simulink subsystem "Subsystem"  (R2024b)
settings: Solver=VariableStepAuto  StartTime=0.0  StopTime=10.0  RelTol=1e-3
settings Model: Creator=samueljoseph  LastModifiedBy=samueljoseph

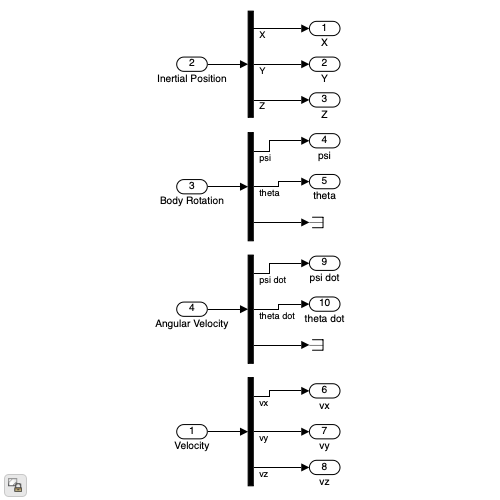
[thumbnail: Simulink's stored preview of the top-level diagram]
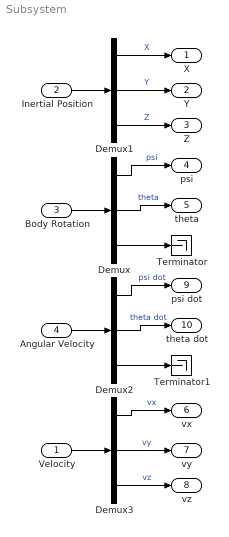
== system Subsystem ==
  Velocity : Inport
  Inertial Position : Inport  Port=2
  Body Rotation : Inport  Port=3
  Angular Velocity : Inport  Port=4
  Demux{,1..3} (4 alike) : Demux  Outputs=3
  Terminator : Terminator
  Terminator1 : Terminator
  X : Outport
  Y : Outport  Port=2
  Z : Outport  Port=3
  psi : Outport  Port=4
  theta : Outport  Port=5
  vx : Outport  Port=6
  vy : Outport  Port=7
  vz : Outport  Port=8
  psi dot : Outport  Port=9
  theta dot : Outport  Port=10
  wires:
  Demux3/3 -> vz/1  "vz"
  Demux3/2 -> vy/1  "vy"
  Demux1/2 -> Y/1  "Y"
  Demux1/1 -> X/1  "X"
  Demux2/3 -> Terminator1/1
  Demux3/1 -> vx/1  "vx"
  Demux2/2 -> theta dot/1  "theta dot"
  Demux1/3 -> Z/1  "Z"
  Demux/2 -> theta/1  "theta"
  Body Rotation/1 -> Demux/1
  Demux/1 -> psi/1  "psi"
  Velocity/1 -> Demux3/1
  Demux2/1 -> psi dot/1  "psi dot"
  Demux/3 -> Terminator/1
  Inertial Position/1 -> Demux1/1
  Angular Velocity/1 -> Demux2/1
